simulink model "QuarterVehicleModel"  (R2022b)
settings: Solver=ode45  StartTime=0.0  StopTime=5  FixedStep=0.001  MaxStep=Ts  RelTol=1e-3  EnableMultiTasking=on
PreLoadFcn:
  | QuarterCarParams
values from neighbouring files (symbols this model uses):
  actuatorDelay = 0.005    [QuarterCarParams.m]
  actuatorPole = 70    [QuarterCarParams.m]
  actuatorSat = 4000    [QuarterCarParams.m]
  g = 9.81    [QuarterCarParams.m]
  J = 1    [QuarterCarParams.m]
  Ki = 100000    [QuarterCarParams.m]
  Kp = 1200    [QuarterCarParams.m]
  lambda_ref = 0.1    [QuarterCarParams.m]
  m = 450    [QuarterCarParams.m]
  roadCoeffs = [1.2801 23.99 0.523 0.03]    [QuarterCarParams.m]
  v0 = 30    [QuarterCarParams.m]
  Wr = 0.32    [QuarterCarParams.m]
undefined symbols (not defined in the file or in its folder): DiscIntNeverNeededParam
libraries: simulink x1
settings Model: Creator=SIMONE  LastModifiedBy=User
settings SolverCC: ZeroCrossAlgorithm=Adaptive  AlgebraicLoopSolver=TrustRegion
settings DataIOCC: SaveFormat=Array  SignalLoggingSaveFormat=ModelDataLogs  SaveOutput=off  SignalLogging=off  DSMLogging=off  SaveTime=off  ReturnWorkspaceOutputs=off  TimeSaveName=t_out
settings OptimizationCC: ExpressionDepthLimit=2147483647  InitFltsAndDblsToZero=on  LifeSpan=inf
settings DebuggingCC: UnderspecifiedInitializationDetection=Classic  MergeDetectMultiDrivingBlocksExec=none  IgnoredZcDiagnostic=none  SolverPrmCheckMsg=warning  FcnCallInpInsideContextMsg=warning  UnconnectedInputMsg=warning  UnconnectedOutputMsg=warning  UnconnectedLineMsg=warning  StateNameClashWarn=warning  SFUnexpectedBacktrackingDiag=warning  SFNoUnconditionalDefaultTransitionDiag=warning  SFExecutionAtInitializationDiag=none  SFMachineParentedDataDiag=warning  ArithmeticOperatorsInVariantConditions=warning
settings HardwareCC: ProdBitPerPointer=32  ProdBitPerSizeT=32  ProdBitPerPtrDiffT=32  ProdLargestAtomicFloat=None  ProdIntDivRoundTo=Undefined  ProdEndianess=Unspecified  ProdWordSize=32  ProdHWDeviceType=32-bit Generic
settings ModelReferenceCC: PropagateSignalLabelsOutOfModel=off
settings SFSimCC: SimUseLocalCustomCode=off  CustomCodeUndefinedFunction=UseInterfaceOnly
settings RTWCC: RTWUseLocalCustomCode=off
settings CodeAppCC: StateflowObjectComments=on
settings GRTTargetCC: TargetLangStandard=C89/C90 (ANSI)  CombineOutputUpdateFcns=off  GRTInterface=on
settings ConfigComp: CovMetricSettings=dw  CovSaveCumulativeToWorkspaceVar=on  CovSaveSingleToWorkspaceVar=on  CovExternalEMLEnable=off

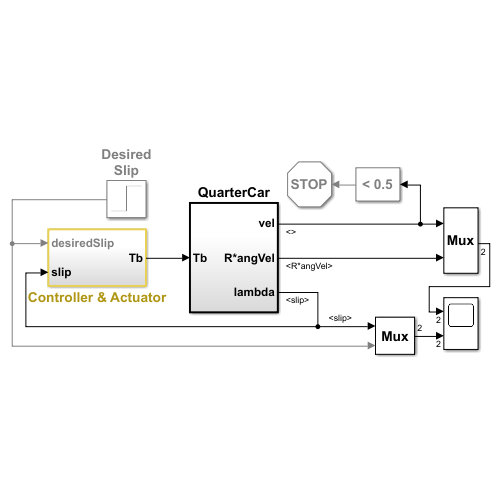
[thumbnail: Simulink's stored preview of the top-level diagram]
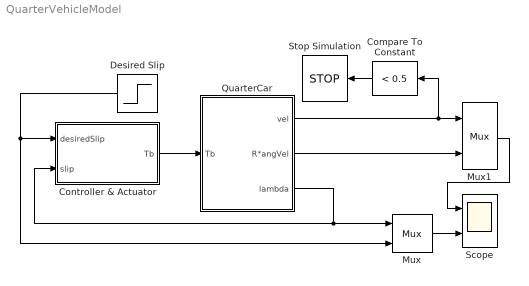
== system QuarterVehicleModel ==
  Compare To Constant : simulink/Logic and Bit Operations/Compare To Constant  relop=<  const=0.5  OutDataTypeStr=boolean
  Controller & Actuator : Subsystem  TreatAsAtomicUnit=on
      settings: MinAlgLoopOccurrences=on
  Desired Slip : Step  Time=0.2  After=lambda_ref  SampleTime=0
  Mux : Mux  Inputs=2
  Mux1 : Mux  Inputs=2
  QuarterCar : Subsystem  TreatAsAtomicUnit=on
      settings: MinAlgLoopOccurrences=on
  Scope : Scope  NumInputPorts=2
  Stop Simulation : Stop
  wires:
  Controller & Actuator/1(Tb) -> QuarterCar/1(Tb)
  Desired Slip/1 -> Mux/2, Controller & Actuator/1(desiredSlip)
  QuarterCar/3(lambda) -> Mux/1, Controller & Actuator/2(slip)
  Mux1/1 -> Scope/1
  Mux/1 -> Scope/2
  QuarterCar/1(vel) -> Mux1/1, Compare To Constant/1
  Compare To Constant/1 -> Stop Simulation/1
  QuarterCar/2(R*angVel) -> Mux1/2

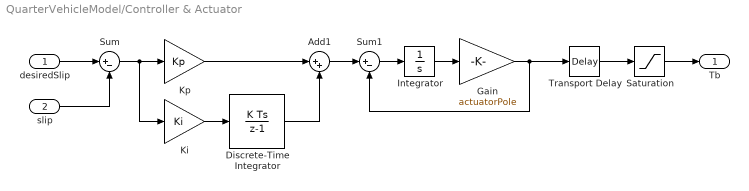
== system QuarterVehicleModel/Controller & Actuator ==
  desiredSlip : Inport
  slip : Inport  Port=2
  Add1 : Sum  Inputs=|++
  Discrete-Time Integrator : DiscreteIntegrator  SampleTime=-1  ICPrevOutput=DiscIntNeverNeededParam  ICPrevScaledInput=DiscIntNeverNeededParam
  Gain : Gain  Gain=actuatorPole
  Integrator : Integrator
  Ki : Gain  Gain=Ki
  Kp : Gain  Gain=Kp
  Saturation : Saturate  UpperLimit=actuatorSat  LowerLimit=0
  Sum : Sum  Inputs=|+-
  Sum1 : Sum  Inputs=|+-
  Transport Delay : TransportDelay  DelayTime=actuatorDelay  BufferSize=10240
  Tb : Outport
  wires:
  Saturation/1 -> Tb/1
  Transport Delay/1 -> Saturation/1
  Ki/1 -> Discrete-Time Integrator/1
  Kp/1 -> Add1/1
  Discrete-Time Integrator/1 -> Add1/2
  Sum/1 -> Ki/1, Kp/1
  desiredSlip/1 -> Sum/1
  slip/1 -> Sum/2
  Integrator/1 -> Gain/1
  Sum1/1 -> Integrator/1
  Add1/1 -> Sum1/1
  Gain/1 -> Transport Delay/1, Sum1/2

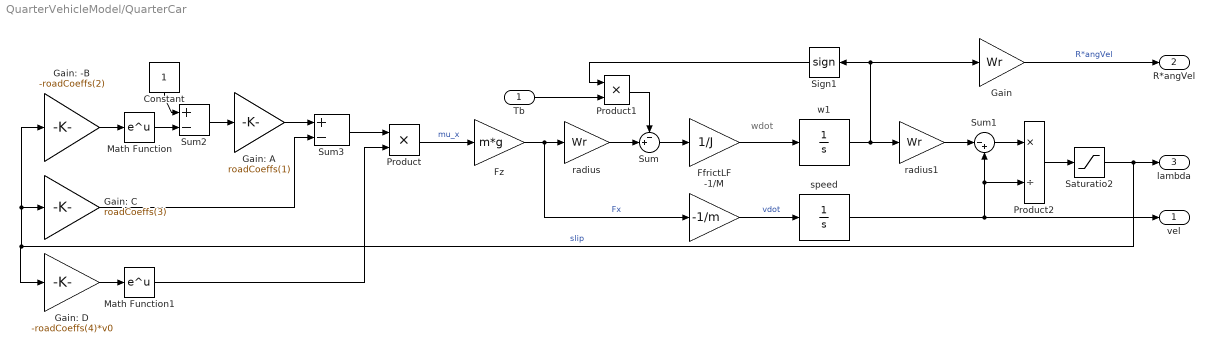
== system QuarterVehicleModel/QuarterCar ==
  note: wdot
  Tb : Inport
  -1/M : Gain  Gain=-1/m  SaturateOnIntegerOverflow=on  OutDataTypeStr=Inherit: Same as input  ParamDataTypeStr=Inherit: Same as input
  Constant : Constant
  FfrictLF : Gain  Gain=1/J  SaturateOnIntegerOverflow=on  OutDataTypeStr=Inherit: Same as input  ParamDataTypeStr=Inherit: Same as input
  Fz : Gain  Gain=m*g  SaturateOnIntegerOverflow=on  OutDataTypeStr=Inherit: Same as input  ParamDataTypeStr=Inherit: Same as input
  Gain : Gain  Gain=Wr
  Gain: -B : Gain  Gain=-roadCoeffs(2)  SaturateOnIntegerOverflow=on  OutDataTypeStr=Inherit: Same as input  ParamDataTypeStr=Inherit: Same as input
  Gain: A : Gain  Gain=roadCoeffs(1)  SaturateOnIntegerOverflow=on  OutDataTypeStr=Inherit: Same as input  ParamDataTypeStr=Inherit: Same as input
  Gain: C : Gain  Gain=roadCoeffs(3)  SaturateOnIntegerOverflow=on  OutDataTypeStr=Inherit: Same as input  ParamDataTypeStr=Inherit: Same as input
  Gain: D : Gain  Gain=-roadCoeffs(4)*v0  SaturateOnIntegerOverflow=on  OutDataTypeStr=Inherit: Same as input  ParamDataTypeStr=Inherit: Same as input
  Math Function : Math  SignedPower=on
  Math Function1 : Math  SignedPower=on
  Product : Product
  Product1 : Product  SaturateOnIntegerOverflow=on  OutDataTypeStr=Inherit: Same as first input
  Product2 : Product  Inputs=*/  SaturateOnIntegerOverflow=on  OutDataTypeStr=Inherit: Same as first input
  Saturatio2 : Saturate  UpperLimit=1  LowerLimit=0
  Sign1 : Signum
  Sum : Sum  Inputs=-+|
  Sum1 : Sum  Inputs=|-+
  Sum2 : Sum  Inputs=+-
  Sum3 : Sum  Inputs=+-
  radius : Gain  Gain=Wr  SaturateOnIntegerOverflow=on  OutDataTypeStr=Inherit: Same as input  ParamDataTypeStr=Inherit: Same as input
  radius1 : Gain  Gain=Wr  SaturateOnIntegerOverflow=on  OutDataTypeStr=Inherit: Same as input  ParamDataTypeStr=Inherit: Same as input
  speed : Integrator  InitialCondition=v0  LimitOutput=on  LowerSaturationLimit=0
  w1 : Integrator  InitialCondition=v0/Wr  LimitOutput=on  LowerSaturationLimit=0
  vel : Outport
  R*angVel : Outport  Port=2
  lambda : Outport  Port=3
  wires:
  -1/M/1 -> speed/1  "vdot"
  Fz/1 -> -1/M/1, radius/1  "Fx"
  Saturatio2/1 -> Gain: -B/1, Gain: C/1, Gain: D/1, lambda/1  "slip"
  FfrictLF/1 -> w1/1
  Sign1/1 -> Product1/1
  Tb/1 -> Product1/2
  w1/1 -> radius1/1, Gain/1, Sign1/1
  Sum/1 -> FfrictLF/1
  Product/1 -> Fz/1  "mu_x"
  radius/1 -> Sum/2
  Product1/1 -> Sum/1
  Gain/1 -> R*angVel/1  "R*angVel"
  Sum1/1 -> Product2/1
  speed/1 -> vel/1, Product2/2, Sum1/2
  Product2/1 -> Saturatio2/1
  radius1/1 -> Sum1/1
  Math Function/1 -> Sum2/2
  Math Function1/1 -> Product/2
  Sum2/1 -> Gain: A/1
  Gain: C/1 -> Sum3/2
  Sum3/1 -> Product/1
  Gain: -B/1 -> Math Function/1
  Gain: A/1 -> Sum3/1
  Gain: D/1 -> Math Function1/1
  Constant/1 -> Sum2/1
